simulink model "c172fg_demo"  (Simulink 4.0)
settings: Solver=ode4  SolverMode=SingleTasking  StartTime=0.0  StopTime=180  FixedStep=0.02  RelTol=1e-3
libraries: simulink_extras x4, aerosimlib x3
settings Model: LastModifiedBy=mariusn  SaveTime=off  SaveOutput=off  LimitDataPoints=off  UnconnectedInputMsg=none  UnconnectedOutputMsg=none  UnconnectedLineMsg=none  BooleanDataType=on

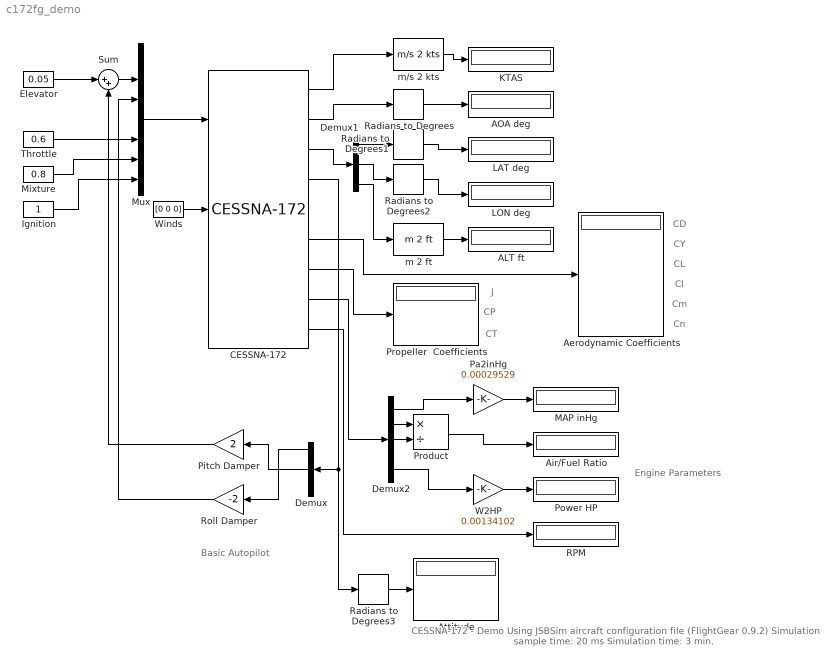
== system c172fg_demo ==
  note: Engine
      |  Parameters
  note: Basic Autopilot
  note: J
  note: CP
  note: CT
  note: CD
  note: CY
  note: CL
  note: Cl
  note: Cm
  note: Cn
  note: CESSNA-172 - Demo
      | Using JSBSim aircraft configuration file
      | (FlightGear 0.9.2)
      | Simulation sample time: 20 ms
      | Simulation time: 3 min.
  ALT ft : Display
      settings: Format=short
  AOA deg : Display
      settings: Format=short
  Aerodynamic Coefficients : Display
      settings: Format=short
  Air/Fuel Ratio : Display
      settings: Format=short
  Attitude : Display
      settings: Format=short
  CESSNA-172 : aerosimlib/FlightGear-Compatible/Complete Aircraft/CESSNA-172  ACName='c172p'  FGPath='c:\flightgear-0.9.2\data'  VelocitiesIni=[60 0 0]'  RatesIni=[0 0 0]'  QuaternionsIni=[1 0 0 0]'  PositionIni=[37.6*pi/180 -122.3*pi/180 2000]'  OmegaIni=2500*pi/30  FuelIni=[50 50]  GndAlt=0  tsamp=0.02
  Demux : Demux  Orientation=left  Outputs=3  BusSelectionMode=off
  Demux1 : Demux  Outputs=3  BusSelectionMode=off
  Demux2 : Demux  Outputs=5  BusSelectionMode=off
  Elevator : Constant  Value=0.05
  Ignition : Constant  Value=1
  KTAS : Display
      settings: Format=short
  LAT deg : Display
      settings: Format=short
  LON deg : Display
      settings: Format=short
  MAP inHg : Display
      settings: Format=short
  Mixture : Constant  Value=0.8
  Mux : Mux  Inputs=7
  Pa2inHg : Gain  Gain=0.00029529  Multiplication=Element-wise(K.*u)  SaturateOnIntegerOverflow=on
  Pitch Damper : Gain  Orientation=left  Gain=2  Multiplication=Element-wise(K.*u)  SaturateOnIntegerOverflow=on
  Power HP : Display
      settings: Format=short
  Product : Product  Inputs=*/  Multiplication=Element-wise(.*)  SaturateOnIntegerOverflow=on
  Propeller  Coefficients : Display
      settings: Format=short
  RPM : Display
      settings: Format=short
  Radians to Degrees{,1..3} (4 alike) : simulink_extras/Transformations/Radians to Degrees
  Roll Damper : Gain  Orientation=left  Gain=-2  Multiplication=Element-wise(K.*u)  SaturateOnIntegerOverflow=on
  Sum : Sum  Inputs=|++  SaturateOnIntegerOverflow=on
  Throttle : Constant  Value=0.6
  W2HP : Gain  Gain=0.00134102  Multiplication=Element-wise(K.*u)  SaturateOnIntegerOverflow=on
  Winds : Constant  Value=[0 0 0]
  m 2 ft : aerosimlib/Unit Conversion/Distance/m 2 ft
  m/s 2 kts : aerosimlib/Unit Conversion/Velocity/m//s 2 kts
  wires:
  Mux/1 -> CESSNA-172/1
  Winds/1 -> CESSNA-172/2
  Throttle/1 -> Mux/5
  Mixture/1 -> Mux/6
  Ignition/1 -> Mux/7
  Elevator/1 -> Sum/1
  Sum/1 -> Mux/2
  Demux/1 -> Roll Damper/1
  Demux/2 -> Pitch Damper/1
  CESSNA-172/4 -> Demux/1, Radians to Degrees3/1
  Pitch Damper/1 -> Sum/2
  Roll Damper/1 -> Mux/3
  m/s 2 kts/1 -> KTAS/1
  CESSNA-172/1 -> m/s 2 kts/1
  CESSNA-172/2 -> Radians to Degrees/1
  Radians to Degrees/1 -> AOA deg/1
  CESSNA-172/3 -> Demux1/1
  Demux1/1 -> Radians to Degrees1/1
  Demux1/2 -> Radians to Degrees2/1
  Radians to Degrees1/1 -> LAT deg/1
  Radians to Degrees2/1 -> LON deg/1
  m 2 ft/1 -> ALT ft/1
  Demux1/3 -> m 2 ft/1
  CESSNA-172/6 -> Aerodynamic Coefficients/1
  CESSNA-172/7 -> Propeller  Coefficients/1
  CESSNA-172/8 -> Demux2/1
  Demux2/1 -> Pa2inHg/1
  Pa2inHg/1 -> MAP inHg/1
  Demux2/2 -> Product/1
  Demux2/3 -> Product/2
  Product/1 -> Air/Fuel Ratio/1
  W2HP/1 -> Power HP/1
  Demux2/5 -> W2HP/1
  CESSNA-172/9 -> RPM/1
  Radians to Degrees3/1 -> Attitude/1
